simulink model "FRNmodel"  (Simulink 7.9)
settings: Solver=VariableStepDiscrete  StartTime=0.0  StopTime=100.0  RelTol=1e-3
libraries: simeventslib x22, FRN_Library x11
(part 1 of 2)
settings Model: Creator=tsprock3  LastModifiedBy=tsprock3
settings DebuggingCC: SimStateOlderReleaseMsg=warning

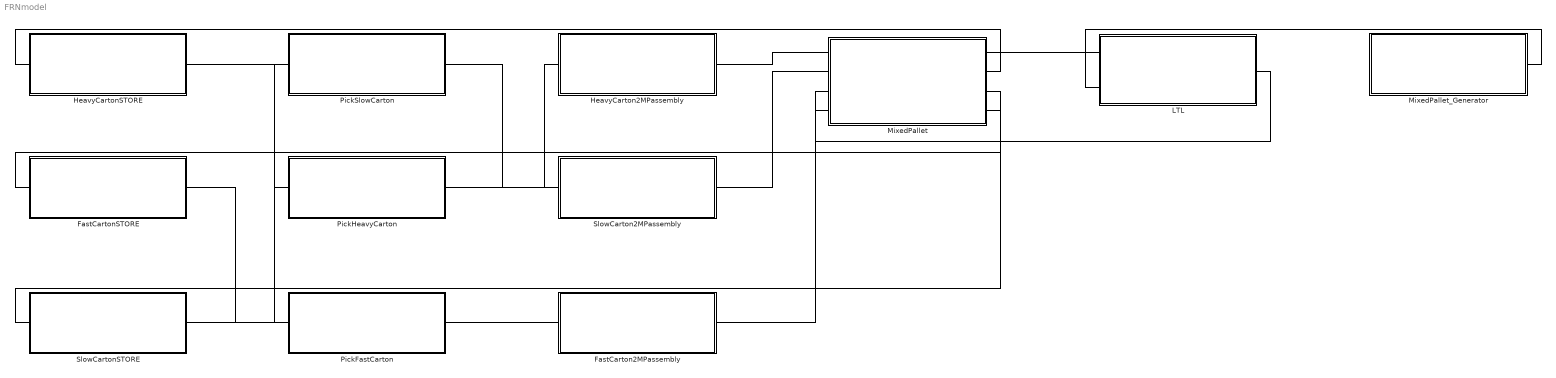
== system FRNmodel ==
  FastCarton2MPassembly : Subsystem
  FastCartonSTORE : Subsystem
  HeavyCarton2MPassembly : Subsystem
  HeavyCartonSTORE : Subsystem
  LTL : Subsystem
  MixedPallet : Subsystem
  MixedPallet_Generator : Subsystem
  PickFastCarton : Subsystem
  PickHeavyCarton : Subsystem
  PickSlowCarton : Subsystem
  SlowCarton2MPassembly : Subsystem
  SlowCartonSTORE : Subsystem
  connections:
  FastCartonSTORE/RConn1 -- PickFastCarton/LConn1
  PickFastCarton/RConn1 -- FastCarton2MPassembly/LConn1
  HeavyCarton2MPassembly/RConn1 -- MixedPallet/LConn1
  MixedPallet/RConn1 -- LTL/LConn1
  PickSlowCarton/RConn1 -- SlowCarton2MPassembly/LConn1
  SlowCarton2MPassembly/RConn1 -- MixedPallet/LConn2
  SlowCartonSTORE/RConn1 -- PickSlowCarton/LConn1
  HeavyCartonSTORE/RConn1 -- PickHeavyCarton/LConn1
  FastCarton2MPassembly/RConn1 -- MixedPallet/LConn3
  PickHeavyCarton/RConn1 -- HeavyCarton2MPassembly/LConn1
  LTL/RConn1 -- MixedPallet/LConn4
  MixedPallet/RConn2 -- HeavyCartonSTORE/LConn1
  MixedPallet/RConn3 -- FastCartonSTORE/LConn1
  MixedPallet/RConn4 -- SlowCartonSTORE/LConn1
  MixedPallet_Generator/RConn1 -- LTL/LConn2

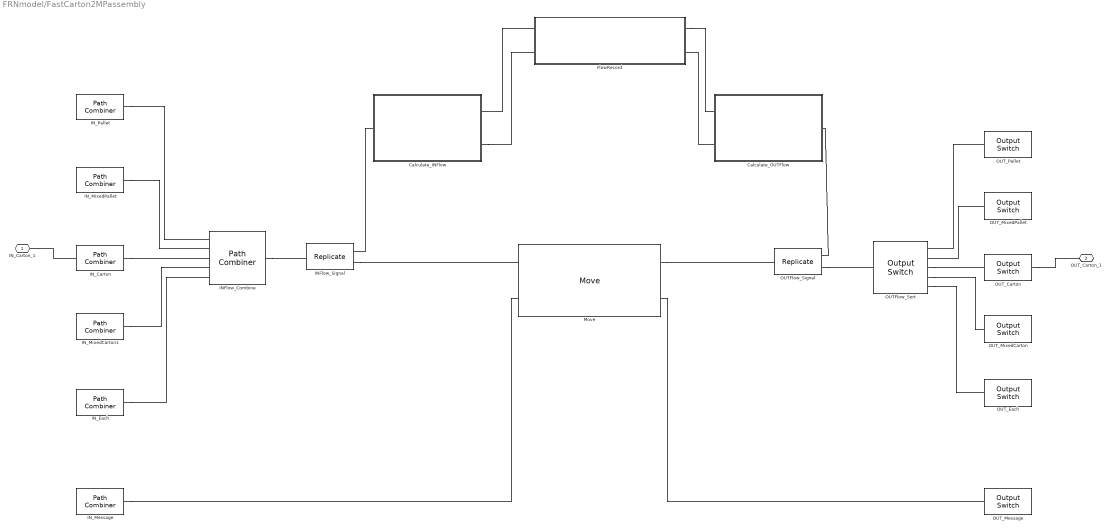
== system FRNmodel/FastCarton2MPassembly ==
  Calculate_INFlow : Subsystem
  Calculate_OUTFlow : Subsystem
  FlowRecord : Subsystem
  INFlow_Combine : PathCombiner  NumberInputPorts=5
  INFlow_Signal : Replicate  NumberOutputPorts=2
  IN_Carton : PathCombiner  NumberInputPorts=1
  IN_Each : PathCombiner  NumberInputPorts=1
  IN_Message : PathCombiner  NumberInputPorts=1
  IN_MixedCarton1 : PathCombiner  NumberInputPorts=1
  IN_MixedPallet : PathCombiner  NumberInputPorts=1
  IN_Pallet : PathCombiner  NumberInputPorts=1
  Move : FRN_Library/Move
  OUTFlow_Signal : Replicate  NumberOutputPorts=2
  OUTFlow_Sort : OutputSwitch  NumberOutputPorts=5  SwitchingCriterion=From attribute  AttributeName=UoH
  OUT_Carton : OutputSwitch  NumberOutputPorts=1
  OUT_Each : OutputSwitch  NumberOutputPorts=1
  OUT_Message : OutputSwitch  NumberOutputPorts=1  SwitchingCriterion=Equiprobable  AttributeName=FlowSource
  OUT_MixedCarton : OutputSwitch  NumberOutputPorts=1
  OUT_MixedPallet : OutputSwitch  NumberOutputPorts=1
  OUT_Pallet : OutputSwitch  NumberOutputPorts=1
  IN_Carton_1 : PMIOPort  Port=1  Side=Left
  OUT_Carton_1 : PMIOPort  Port=2  Side=Right
  connections:
  INFlow_Signal/RConn2 -- Move/LConn1
  IN_MixedCarton1/RConn1 -- INFlow_Combine/LConn4
  IN_MixedPallet/RConn1 -- INFlow_Combine/LConn2
  OUTFlow_Sort/RConn4 -- OUT_MixedCarton/LConn1
  OUT_MixedPallet/LConn1 -- OUTFlow_Sort/RConn2
  Move/RConn2 -- OUT_Message/LConn1
  IN_Message/RConn1 -- Move/LConn2
  OUTFlow_Sort/RConn5 -- OUT_Each/LConn1
  OUTFlow_Sort/RConn3 -- OUT_Carton/LConn1
  OUT_Pallet/LConn1 -- OUTFlow_Sort/RConn1
  OUTFlow_Signal/RConn2 -- OUTFlow_Sort/LConn1
  IN_Each/RConn1 -- INFlow_Combine/LConn5
  IN_Carton/RConn1 -- INFlow_Combine/LConn3
  IN_Pallet/RConn1 -- INFlow_Combine/LConn1
  INFlow_Combine/RConn1 -- INFlow_Signal/LConn1
  OUTFlow_Signal/RConn1 -- Calculate_OUTFlow/RConn1
  Move/RConn1 -- OUTFlow_Signal/LConn1
  Calculate_OUTFlow/LConn2 -- FlowRecord/LConn2
  FlowRecord/LConn1 -- Calculate_OUTFlow/LConn1
  Calculate_INFlow/RConn2 -- FlowRecord/RConn2
  FlowRecord/RConn1 -- Calculate_INFlow/RConn1
  Calculate_INFlow/LConn1 -- INFlow_Signal/RConn1
  IN_Carton/LConn1 -- IN_Carton_1/RConn1
  OUT_Carton/RConn1 -- OUT_Carton_1/RConn1

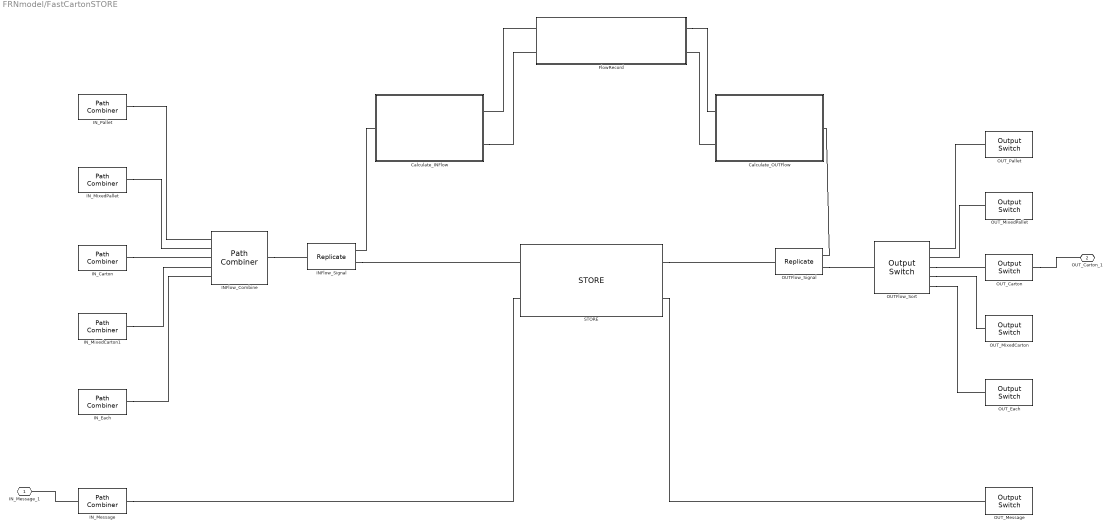
== system FRNmodel/FastCartonSTORE ==
  Calculate_INFlow : Subsystem
  Calculate_OUTFlow : Subsystem
  FlowRecord : Subsystem
  INFlow_Combine : PathCombiner  NumberInputPorts=5
  INFlow_Signal : Replicate  NumberOutputPorts=2
  IN_Carton : PathCombiner  NumberInputPorts=1
  IN_Each : PathCombiner  NumberInputPorts=1
  IN_Message : PathCombiner  NumberInputPorts=1
  IN_MixedCarton1 : PathCombiner  NumberInputPorts=1
  IN_MixedPallet : PathCombiner  NumberInputPorts=1
  IN_Pallet : PathCombiner  NumberInputPorts=1
  OUTFlow_Signal : Replicate  NumberOutputPorts=2
  OUTFlow_Sort : OutputSwitch  NumberOutputPorts=5  SwitchingCriterion=From attribute  AttributeName=UoH
  OUT_Carton : OutputSwitch  NumberOutputPorts=1
  OUT_Each : OutputSwitch  NumberOutputPorts=1
  OUT_Message : OutputSwitch  NumberOutputPorts=1  SwitchingCriterion=Equiprobable  AttributeName=FlowSource
  OUT_MixedCarton : OutputSwitch  NumberOutputPorts=1
  OUT_MixedPallet : OutputSwitch  NumberOutputPorts=1
  OUT_Pallet : OutputSwitch  NumberOutputPorts=1
  STORE : FRN_Library/STORE
  IN_Message_1 : PMIOPort  Port=1  Side=Left
  OUT_Carton_1 : PMIOPort  Port=2  Side=Right
  connections:
  INFlow_Signal/RConn2 -- STORE/LConn1
  IN_MixedCarton1/RConn1 -- INFlow_Combine/LConn4
  IN_MixedPallet/RConn1 -- INFlow_Combine/LConn2
  OUTFlow_Sort/RConn4 -- OUT_MixedCarton/LConn1
  OUT_MixedPallet/LConn1 -- OUTFlow_Sort/RConn2
  STORE/RConn2 -- OUT_Message/LConn1
  IN_Message/RConn1 -- STORE/LConn2
  OUTFlow_Sort/RConn5 -- OUT_Each/LConn1
  OUTFlow_Sort/RConn3 -- OUT_Carton/LConn1
  OUT_Pallet/LConn1 -- OUTFlow_Sort/RConn1
  OUTFlow_Signal/RConn2 -- OUTFlow_Sort/LConn1
  IN_Each/RConn1 -- INFlow_Combine/LConn5
  IN_Carton/RConn1 -- INFlow_Combine/LConn3
  IN_Pallet/RConn1 -- INFlow_Combine/LConn1
  INFlow_Combine/RConn1 -- INFlow_Signal/LConn1
  OUTFlow_Signal/RConn1 -- Calculate_OUTFlow/RConn1
  STORE/RConn1 -- OUTFlow_Signal/LConn1
  Calculate_OUTFlow/LConn2 -- FlowRecord/LConn2
  FlowRecord/LConn1 -- Calculate_OUTFlow/LConn1
  Calculate_INFlow/RConn2 -- FlowRecord/RConn2
  FlowRecord/RConn1 -- Calculate_INFlow/RConn1
  Calculate_INFlow/LConn1 -- INFlow_Signal/RConn1
  IN_Message/LConn1 -- IN_Message_1/RConn1
  OUT_Carton/RConn1 -- OUT_Carton_1/RConn1

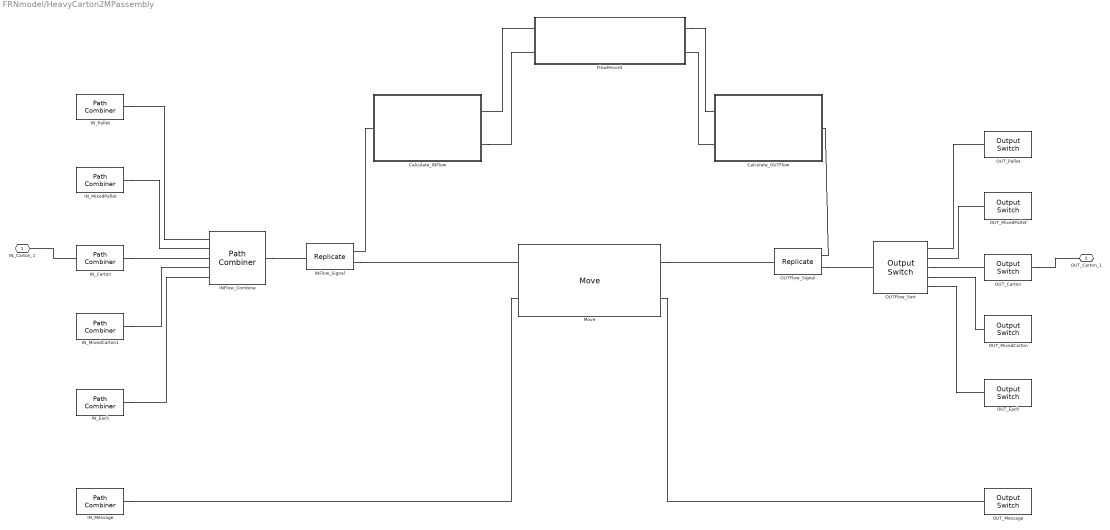
== system FRNmodel/HeavyCarton2MPassembly ==
  Calculate_INFlow : Subsystem
  Calculate_OUTFlow : Subsystem
  FlowRecord : Subsystem
  INFlow_Combine : PathCombiner  NumberInputPorts=5
  INFlow_Signal : Replicate  NumberOutputPorts=2
  IN_Carton : PathCombiner  NumberInputPorts=1
  IN_Each : PathCombiner  NumberInputPorts=1
  IN_Message : PathCombiner  NumberInputPorts=1
  IN_MixedCarton1 : PathCombiner  NumberInputPorts=1
  IN_MixedPallet : PathCombiner  NumberInputPorts=1
  IN_Pallet : PathCombiner  NumberInputPorts=1
  Move : FRN_Library/Move
  OUTFlow_Signal : Replicate  NumberOutputPorts=2
  OUTFlow_Sort : OutputSwitch  NumberOutputPorts=5  SwitchingCriterion=From attribute  AttributeName=UoH
  OUT_Carton : OutputSwitch  NumberOutputPorts=1
  OUT_Each : OutputSwitch  NumberOutputPorts=1
  OUT_Message : OutputSwitch  NumberOutputPorts=1  SwitchingCriterion=Equiprobable  AttributeName=FlowSource
  OUT_MixedCarton : OutputSwitch  NumberOutputPorts=1
  OUT_MixedPallet : OutputSwitch  NumberOutputPorts=1
  OUT_Pallet : OutputSwitch  NumberOutputPorts=1
  IN_Carton_1 : PMIOPort  Port=1  Side=Left
  OUT_Carton_1 : PMIOPort  Port=2  Side=Right
  connections:
  INFlow_Signal/RConn2 -- Move/LConn1
  IN_MixedCarton1/RConn1 -- INFlow_Combine/LConn4
  IN_MixedPallet/RConn1 -- INFlow_Combine/LConn2
  OUTFlow_Sort/RConn4 -- OUT_MixedCarton/LConn1
  OUT_MixedPallet/LConn1 -- OUTFlow_Sort/RConn2
  Move/RConn2 -- OUT_Message/LConn1
  IN_Message/RConn1 -- Move/LConn2
  OUTFlow_Sort/RConn5 -- OUT_Each/LConn1
  OUTFlow_Sort/RConn3 -- OUT_Carton/LConn1
  OUT_Pallet/LConn1 -- OUTFlow_Sort/RConn1
  OUTFlow_Signal/RConn2 -- OUTFlow_Sort/LConn1
  IN_Each/RConn1 -- INFlow_Combine/LConn5
  IN_Carton/RConn1 -- INFlow_Combine/LConn3
  IN_Pallet/RConn1 -- INFlow_Combine/LConn1
  INFlow_Combine/RConn1 -- INFlow_Signal/LConn1
  OUTFlow_Signal/RConn1 -- Calculate_OUTFlow/RConn1
  Move/RConn1 -- OUTFlow_Signal/LConn1
  Calculate_OUTFlow/LConn2 -- FlowRecord/LConn2
  FlowRecord/LConn1 -- Calculate_OUTFlow/LConn1
  Calculate_INFlow/RConn2 -- FlowRecord/RConn2
  FlowRecord/RConn1 -- Calculate_INFlow/RConn1
  Calculate_INFlow/LConn1 -- INFlow_Signal/RConn1
  IN_Carton/LConn1 -- IN_Carton_1/RConn1
  OUT_Carton/RConn1 -- OUT_Carton_1/RConn1

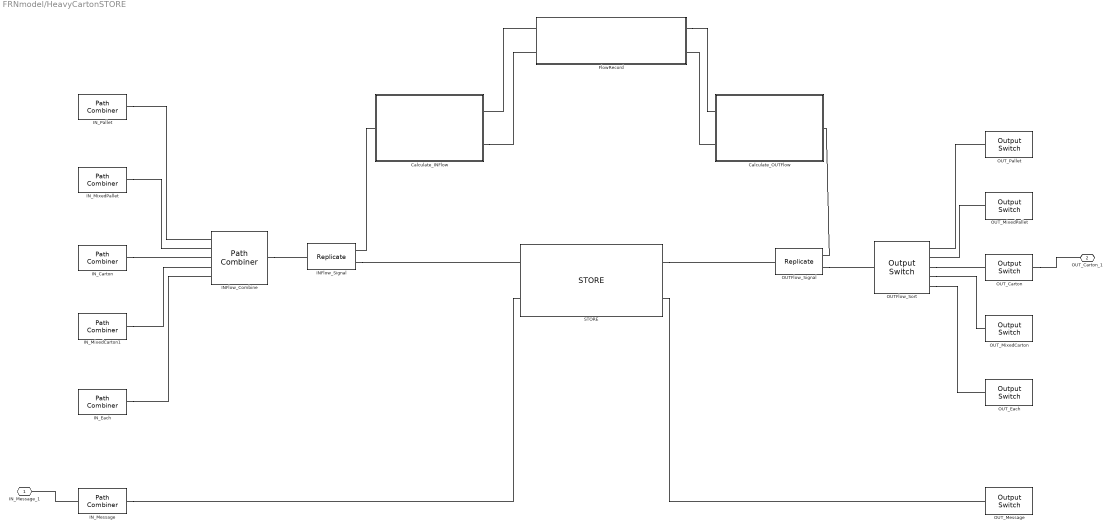
== system FRNmodel/HeavyCartonSTORE ==
  Calculate_INFlow : Subsystem
  Calculate_OUTFlow : Subsystem
  FlowRecord : Subsystem
  INFlow_Combine : PathCombiner  NumberInputPorts=5
  INFlow_Signal : Replicate  NumberOutputPorts=2
  IN_Carton : PathCombiner  NumberInputPorts=1
  IN_Each : PathCombiner  NumberInputPorts=1
  IN_Message : PathCombiner  NumberInputPorts=1
  IN_MixedCarton1 : PathCombiner  NumberInputPorts=1
  IN_MixedPallet : PathCombiner  NumberInputPorts=1
  IN_Pallet : PathCombiner  NumberInputPorts=1
  OUTFlow_Signal : Replicate  NumberOutputPorts=2
  OUTFlow_Sort : OutputSwitch  NumberOutputPorts=5  SwitchingCriterion=From attribute  AttributeName=UoH
  OUT_Carton : OutputSwitch  NumberOutputPorts=1
  OUT_Each : OutputSwitch  NumberOutputPorts=1
  OUT_Message : OutputSwitch  NumberOutputPorts=1  SwitchingCriterion=Equiprobable  AttributeName=FlowSource
  OUT_MixedCarton : OutputSwitch  NumberOutputPorts=1
  OUT_MixedPallet : OutputSwitch  NumberOutputPorts=1
  OUT_Pallet : OutputSwitch  NumberOutputPorts=1
  STORE : FRN_Library/STORE
  IN_Message_1 : PMIOPort  Port=1  Side=Left
  OUT_Carton_1 : PMIOPort  Port=2  Side=Right
  connections:
  INFlow_Signal/RConn2 -- STORE/LConn1
  IN_MixedCarton1/RConn1 -- INFlow_Combine/LConn4
  IN_MixedPallet/RConn1 -- INFlow_Combine/LConn2
  OUTFlow_Sort/RConn4 -- OUT_MixedCarton/LConn1
  OUT_MixedPallet/LConn1 -- OUTFlow_Sort/RConn2
  STORE/RConn2 -- OUT_Message/LConn1
  IN_Message/RConn1 -- STORE/LConn2
  OUTFlow_Sort/RConn5 -- OUT_Each/LConn1
  OUTFlow_Sort/RConn3 -- OUT_Carton/LConn1
  OUT_Pallet/LConn1 -- OUTFlow_Sort/RConn1
  OUTFlow_Signal/RConn2 -- OUTFlow_Sort/LConn1
  IN_Each/RConn1 -- INFlow_Combine/LConn5
  IN_Carton/RConn1 -- INFlow_Combine/LConn3
  IN_Pallet/RConn1 -- INFlow_Combine/LConn1
  INFlow_Combine/RConn1 -- INFlow_Signal/LConn1
  OUTFlow_Signal/RConn1 -- Calculate_OUTFlow/RConn1
  STORE/RConn1 -- OUTFlow_Signal/LConn1
  Calculate_OUTFlow/LConn2 -- FlowRecord/LConn2
  FlowRecord/LConn1 -- Calculate_OUTFlow/LConn1
  Calculate_INFlow/RConn2 -- FlowRecord/RConn2
  FlowRecord/RConn1 -- Calculate_INFlow/RConn1
  Calculate_INFlow/LConn1 -- INFlow_Signal/RConn1
  IN_Message/LConn1 -- IN_Message_1/RConn1
  OUT_Carton/RConn1 -- OUT_Carton_1/RConn1

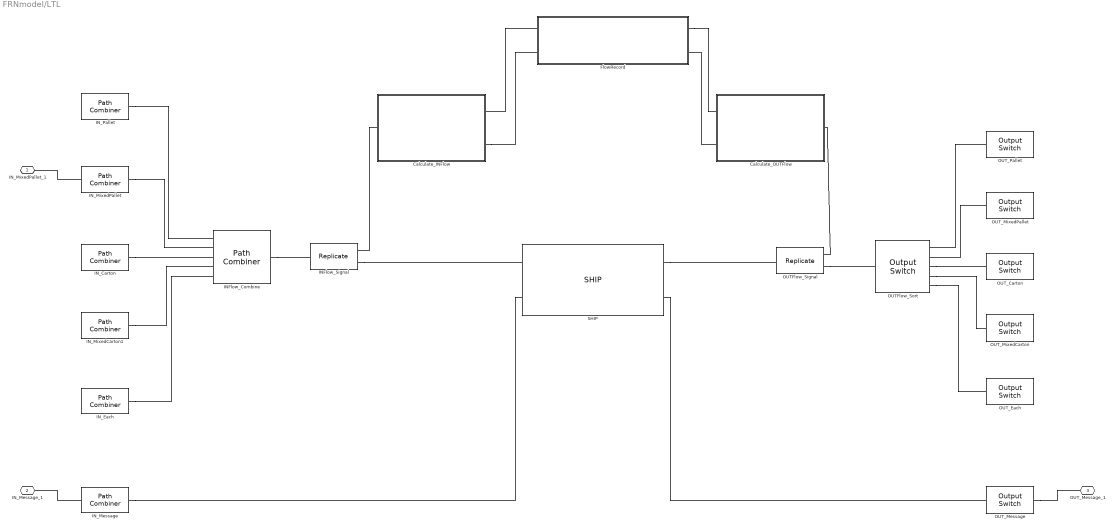
== system FRNmodel/LTL ==
  Calculate_INFlow : Subsystem
  Calculate_OUTFlow : Subsystem
  FlowRecord : Subsystem
  INFlow_Combine : PathCombiner  NumberInputPorts=5
  INFlow_Signal : Replicate  NumberOutputPorts=2
  IN_Carton : PathCombiner  NumberInputPorts=1
  IN_Each : PathCombiner  NumberInputPorts=1
  IN_Message : PathCombiner  NumberInputPorts=1
  IN_MixedCarton1 : PathCombiner  NumberInputPorts=1
  IN_MixedPallet : PathCombiner  NumberInputPorts=1
  IN_Pallet : PathCombiner  NumberInputPorts=1
  OUTFlow_Signal : Replicate  NumberOutputPorts=2
  OUTFlow_Sort : OutputSwitch  NumberOutputPorts=5  SwitchingCriterion=From attribute  AttributeName=UoH
  OUT_Carton : OutputSwitch  NumberOutputPorts=1
  OUT_Each : OutputSwitch  NumberOutputPorts=1
  OUT_Message : OutputSwitch  NumberOutputPorts=1  SwitchingCriterion=Equiprobable  AttributeName=FlowSource
  OUT_MixedCarton : OutputSwitch  NumberOutputPorts=1
  OUT_MixedPallet : OutputSwitch  NumberOutputPorts=1
  OUT_Pallet : OutputSwitch  NumberOutputPorts=1
  SHIP : FRN_Library/SHIP
  IN_MixedPallet_1 : PMIOPort  Port=1  Side=Left
  IN_Message_1 : PMIOPort  Port=2  Side=Left
  OUT_Message_1 : PMIOPort  Port=3  Side=Right
  connections:
  INFlow_Signal/RConn2 -- SHIP/LConn1
  IN_MixedCarton1/RConn1 -- INFlow_Combine/LConn4
  IN_MixedPallet/RConn1 -- INFlow_Combine/LConn2
  OUTFlow_Sort/RConn4 -- OUT_MixedCarton/LConn1
  OUT_MixedPallet/LConn1 -- OUTFlow_Sort/RConn2
  SHIP/RConn2 -- OUT_Message/LConn1
  IN_Message/RConn1 -- SHIP/LConn2
  OUTFlow_Sort/RConn5 -- OUT_Each/LConn1
  OUTFlow_Sort/RConn3 -- OUT_Carton/LConn1
  OUT_Pallet/LConn1 -- OUTFlow_Sort/RConn1
  OUTFlow_Signal/RConn2 -- OUTFlow_Sort/LConn1
  IN_Each/RConn1 -- INFlow_Combine/LConn5
  IN_Carton/RConn1 -- INFlow_Combine/LConn3
  IN_Pallet/RConn1 -- INFlow_Combine/LConn1
  INFlow_Combine/RConn1 -- INFlow_Signal/LConn1
  OUTFlow_Signal/RConn1 -- Calculate_OUTFlow/RConn1
  SHIP/RConn1 -- OUTFlow_Signal/LConn1
  Calculate_OUTFlow/LConn2 -- FlowRecord/LConn2
  FlowRecord/LConn1 -- Calculate_OUTFlow/LConn1
  Calculate_INFlow/RConn2 -- FlowRecord/RConn2
  FlowRecord/RConn1 -- Calculate_INFlow/RConn1
  Calculate_INFlow/LConn1 -- INFlow_Signal/RConn1
  IN_MixedPallet/LConn1 -- IN_MixedPallet_1/RConn1
  IN_Message/LConn1 -- IN_Message_1/RConn1
  OUT_Message/RConn1 -- OUT_Message_1/RConn1

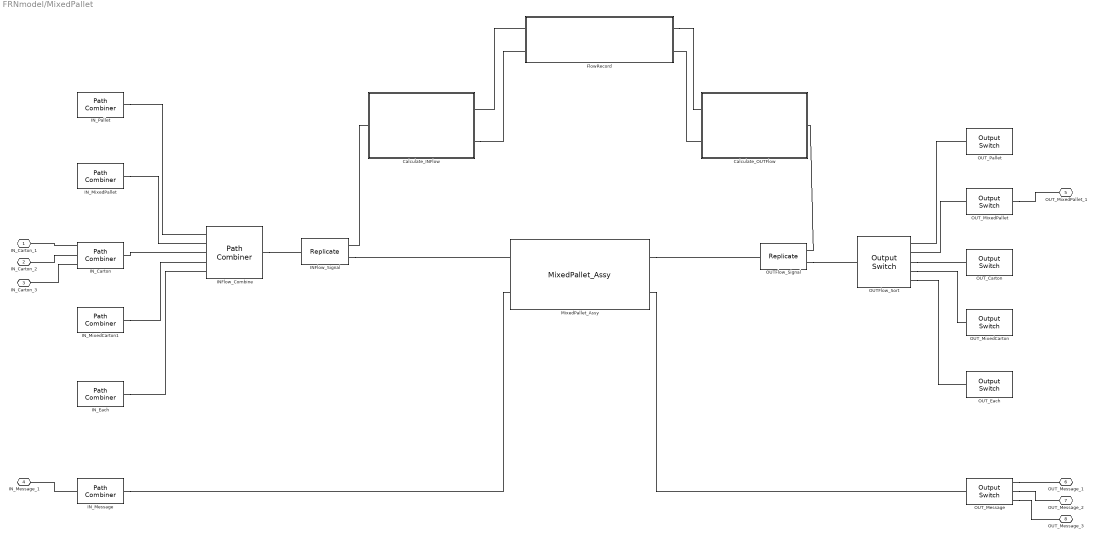
== system FRNmodel/MixedPallet ==
  Calculate_INFlow : Subsystem
  Calculate_OUTFlow : Subsystem
  FlowRecord : Subsystem
  INFlow_Combine : PathCombiner  NumberInputPorts=5
  INFlow_Signal : Replicate  NumberOutputPorts=2
  IN_Carton : PathCombiner
  IN_Each : PathCombiner  NumberInputPorts=1
  IN_Message : PathCombiner  NumberInputPorts=1
  IN_MixedCarton1 : PathCombiner  NumberInputPorts=1
  IN_MixedPallet : PathCombiner  NumberInputPorts=1
  IN_Pallet : PathCombiner  NumberInputPorts=1
  MixedPallet_Assy : FRN_Library/MixedPallet_Assy
  OUTFlow_Signal : Replicate  NumberOutputPorts=2
  OUTFlow_Sort : OutputSwitch  NumberOutputPorts=5  SwitchingCriterion=From attribute  AttributeName=UoH
  OUT_Carton : OutputSwitch  NumberOutputPorts=1
  OUT_Each : OutputSwitch  NumberOutputPorts=1
  OUT_Message : OutputSwitch  SwitchingCriterion=Equiprobable  AttributeName=FlowSource
  OUT_MixedCarton : OutputSwitch  NumberOutputPorts=1
  OUT_MixedPallet : OutputSwitch  NumberOutputPorts=1
  OUT_Pallet : OutputSwitch  NumberOutputPorts=1
  IN_Carton_1 : PMIOPort  Port=1  Side=Left
  IN_Carton_2 : PMIOPort  Port=2  Side=Left
  IN_Carton_3 : PMIOPort  Port=3  Side=Left
  IN_Message_1 : PMIOPort  Port=4  Side=Left
  OUT_MixedPallet_1 : PMIOPort  Port=5  Side=Right
  OUT_Message_1 : PMIOPort  Port=6  Side=Right
  OUT_Message_2 : PMIOPort  Port=7  Side=Right
  OUT_Message_3 : PMIOPort  Port=8  Side=Right
  connections:
  INFlow_Signal/RConn2 -- MixedPallet_Assy/LConn1
  IN_MixedCarton1/RConn1 -- INFlow_Combine/LConn4
  IN_MixedPallet/RConn1 -- INFlow_Combine/LConn2
  OUTFlow_Sort/RConn4 -- OUT_MixedCarton/LConn1
  OUT_MixedPallet/LConn1 -- OUTFlow_Sort/RConn2
  MixedPallet_Assy/RConn2 -- OUT_Message/LConn1
  IN_Message/RConn1 -- MixedPallet_Assy/LConn2
  OUTFlow_Sort/RConn5 -- OUT_Each/LConn1
  OUTFlow_Sort/RConn3 -- OUT_Carton/LConn1
  OUT_Pallet/LConn1 -- OUTFlow_Sort/RConn1
  OUTFlow_Signal/RConn2 -- OUTFlow_Sort/LConn1
  IN_Each/RConn1 -- INFlow_Combine/LConn5
  IN_Carton/RConn1 -- INFlow_Combine/LConn3
  IN_Pallet/RConn1 -- INFlow_Combine/LConn1
  INFlow_Combine/RConn1 -- INFlow_Signal/LConn1
  OUTFlow_Signal/RConn1 -- Calculate_OUTFlow/RConn1
  MixedPallet_Assy/RConn1 -- OUTFlow_Signal/LConn1
  Calculate_OUTFlow/LConn2 -- FlowRecord/LConn2
  FlowRecord/LConn1 -- Calculate_OUTFlow/LConn1
  Calculate_INFlow/RConn2 -- FlowRecord/RConn2
  FlowRecord/RConn1 -- Calculate_INFlow/RConn1
  Calculate_INFlow/LConn1 -- INFlow_Signal/RConn1
  IN_Carton/LConn1 -- IN_Carton_1/RConn1
  IN_Carton/LConn2 -- IN_Carton_2/RConn1
  IN_Carton/LConn3 -- IN_Carton_3/RConn1
  IN_Message/LConn1 -- IN_Message_1/RConn1
  OUT_MixedPallet/RConn1 -- OUT_MixedPallet_1/RConn1
  OUT_Message/RConn1 -- OUT_Message_1/RConn1
  OUT_Message/RConn2 -- OUT_Message_2/RConn1
  OUT_Message/RConn3 -- OUT_Message_3/RConn1

== system FRNmodel/MixedPallet_Generator ==
  OUT_Message : OutputSwitch  NumberOutputPorts=1
  Set Attribute : SetAttribute  AttributeName=UoH|CartonQuantity  AttributeFrom=Dialog|Dialog  AttributeValue=3|100  AttributeTreatAsVector=1|1  EvaluatedAttributeValue={3;100}
  Time-Based Entity Generator : TimeBasedEntityGenerator
  OUT_Message_1 : PMIOPort  Port=1  Side=Right
  connections:
  Set Attribute/RConn1 -- OUT_Message/LConn1
  Time-Based Entity Generator/RConn1 -- Set Attribute/LConn1
  OUT_Message/RConn1 -- OUT_Message_1/RConn1

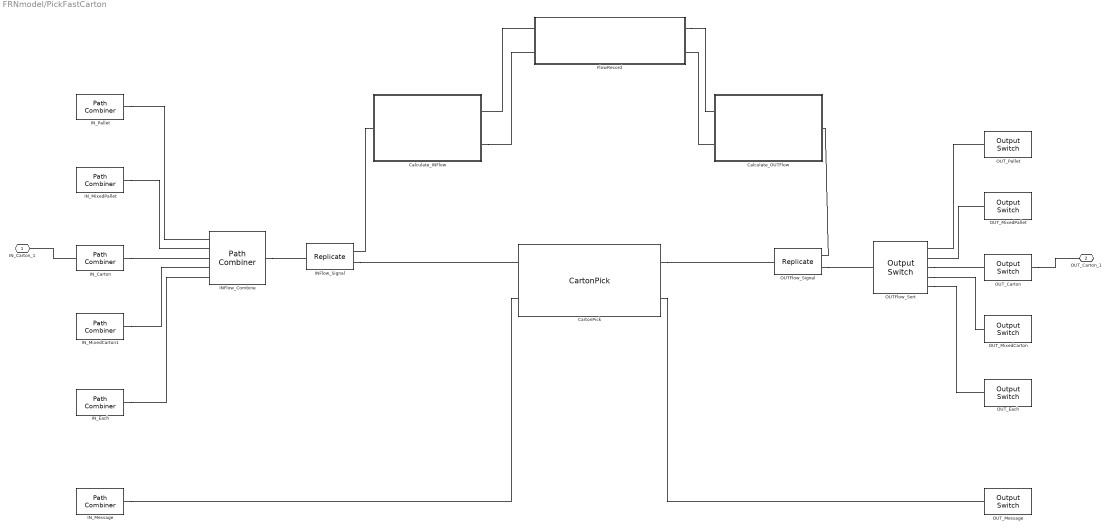
== system FRNmodel/PickFastCarton ==
  Calculate_INFlow : Subsystem
  Calculate_OUTFlow : Subsystem
  CartonPick : FRN_Library/CartonPick
  FlowRecord : Subsystem
  INFlow_Combine : PathCombiner  NumberInputPorts=5
  INFlow_Signal : Replicate  NumberOutputPorts=2
  IN_Carton : PathCombiner  NumberInputPorts=1
  IN_Each : PathCombiner  NumberInputPorts=1
  IN_Message : PathCombiner  NumberInputPorts=1
  IN_MixedCarton1 : PathCombiner  NumberInputPorts=1
  IN_MixedPallet : PathCombiner  NumberInputPorts=1
  IN_Pallet : PathCombiner  NumberInputPorts=1
  OUTFlow_Signal : Replicate  NumberOutputPorts=2
  OUTFlow_Sort : OutputSwitch  NumberOutputPorts=5  SwitchingCriterion=From attribute  AttributeName=UoH
  OUT_Carton : OutputSwitch  NumberOutputPorts=1
  OUT_Each : OutputSwitch  NumberOutputPorts=1
  OUT_Message : OutputSwitch  NumberOutputPorts=1  SwitchingCriterion=Equiprobable  AttributeName=FlowSource
  OUT_MixedCarton : OutputSwitch  NumberOutputPorts=1
  OUT_MixedPallet : OutputSwitch  NumberOutputPorts=1
  OUT_Pallet : OutputSwitch  NumberOutputPorts=1
  IN_Carton_1 : PMIOPort  Port=1  Side=Left
  OUT_Carton_1 : PMIOPort  Port=2  Side=Right
  connections:
  INFlow_Signal/RConn2 -- CartonPick/LConn1
  IN_MixedCarton1/RConn1 -- INFlow_Combine/LConn4
  IN_MixedPallet/RConn1 -- INFlow_Combine/LConn2
  OUTFlow_Sort/RConn4 -- OUT_MixedCarton/LConn1
  OUT_MixedPallet/LConn1 -- OUTFlow_Sort/RConn2
  CartonPick/RConn2 -- OUT_Message/LConn1
  IN_Message/RConn1 -- CartonPick/LConn2
  OUTFlow_Sort/RConn5 -- OUT_Each/LConn1
  OUTFlow_Sort/RConn3 -- OUT_Carton/LConn1
  OUT_Pallet/LConn1 -- OUTFlow_Sort/RConn1
  OUTFlow_Signal/RConn2 -- OUTFlow_Sort/LConn1
  IN_Each/RConn1 -- INFlow_Combine/LConn5
  IN_Carton/RConn1 -- INFlow_Combine/LConn3
  IN_Pallet/RConn1 -- INFlow_Combine/LConn1
  INFlow_Combine/RConn1 -- INFlow_Signal/LConn1
  OUTFlow_Signal/RConn1 -- Calculate_OUTFlow/RConn1
  CartonPick/RConn1 -- OUTFlow_Signal/LConn1
  Calculate_OUTFlow/LConn2 -- FlowRecord/LConn2
  FlowRecord/LConn1 -- Calculate_OUTFlow/LConn1
  Calculate_INFlow/RConn2 -- FlowRecord/RConn2
  FlowRecord/RConn1 -- Calculate_INFlow/RConn1
  Calculate_INFlow/LConn1 -- INFlow_Signal/RConn1
  IN_Carton/LConn1 -- IN_Carton_1/RConn1
  OUT_Carton/RConn1 -- OUT_Carton_1/RConn1

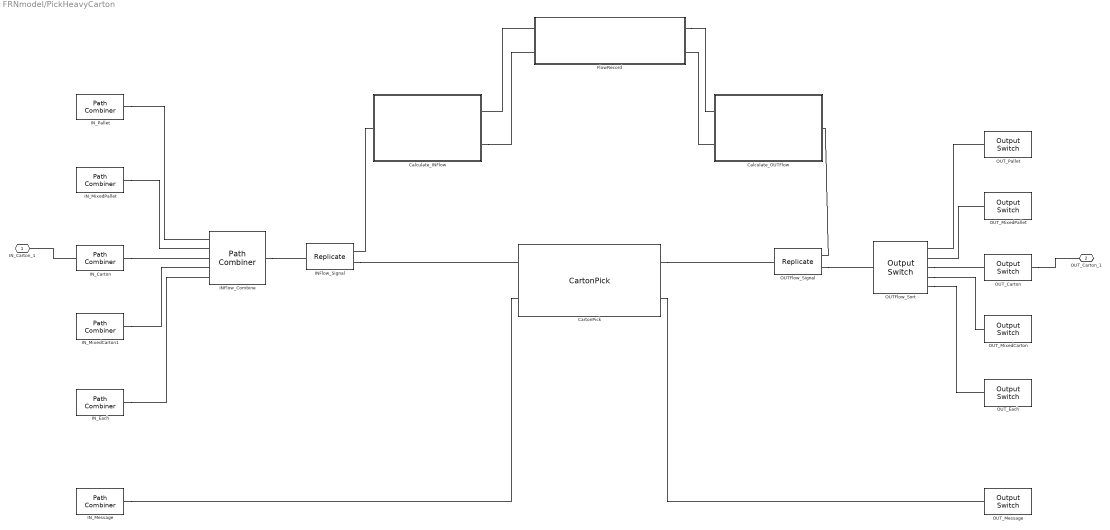
== system FRNmodel/PickHeavyCarton ==
  Calculate_INFlow : Subsystem
  Calculate_OUTFlow : Subsystem
  CartonPick : FRN_Library/CartonPick
  FlowRecord : Subsystem
  INFlow_Combine : PathCombiner  NumberInputPorts=5
  INFlow_Signal : Replicate  NumberOutputPorts=2
  IN_Carton : PathCombiner  NumberInputPorts=1
  IN_Each : PathCombiner  NumberInputPorts=1
  IN_Message : PathCombiner  NumberInputPorts=1
  IN_MixedCarton1 : PathCombiner  NumberInputPorts=1
  IN_MixedPallet : PathCombiner  NumberInputPorts=1
  IN_Pallet : PathCombiner  NumberInputPorts=1
  OUTFlow_Signal : Replicate  NumberOutputPorts=2
  OUTFlow_Sort : OutputSwitch  NumberOutputPorts=5  SwitchingCriterion=From attribute  AttributeName=UoH
  OUT_Carton : OutputSwitch  NumberOutputPorts=1
  OUT_Each : OutputSwitch  NumberOutputPorts=1
  OUT_Message : OutputSwitch  NumberOutputPorts=1  SwitchingCriterion=Equiprobable  AttributeName=FlowSource
  OUT_MixedCarton : OutputSwitch  NumberOutputPorts=1
  OUT_MixedPallet : OutputSwitch  NumberOutputPorts=1
  OUT_Pallet : OutputSwitch  NumberOutputPorts=1
  IN_Carton_1 : PMIOPort  Port=1  Side=Left
  OUT_Carton_1 : PMIOPort  Port=2  Side=Right
  connections:
  INFlow_Signal/RConn2 -- CartonPick/LConn1
  IN_MixedCarton1/RConn1 -- INFlow_Combine/LConn4
  IN_MixedPallet/RConn1 -- INFlow_Combine/LConn2
  OUTFlow_Sort/RConn4 -- OUT_MixedCarton/LConn1
  OUT_MixedPallet/LConn1 -- OUTFlow_Sort/RConn2
  CartonPick/RConn2 -- OUT_Message/LConn1
  IN_Message/RConn1 -- CartonPick/LConn2
  OUTFlow_Sort/RConn5 -- OUT_Each/LConn1
  OUTFlow_Sort/RConn3 -- OUT_Carton/LConn1
  OUT_Pallet/LConn1 -- OUTFlow_Sort/RConn1
  OUTFlow_Signal/RConn2 -- OUTFlow_Sort/LConn1
  IN_Each/RConn1 -- INFlow_Combine/LConn5
  IN_Carton/RConn1 -- INFlow_Combine/LConn3
  IN_Pallet/RConn1 -- INFlow_Combine/LConn1
  INFlow_Combine/RConn1 -- INFlow_Signal/LConn1
  OUTFlow_Signal/RConn1 -- Calculate_OUTFlow/RConn1
  CartonPick/RConn1 -- OUTFlow_Signal/LConn1
  Calculate_OUTFlow/LConn2 -- FlowRecord/LConn2
  FlowRecord/LConn1 -- Calculate_OUTFlow/LConn1
  Calculate_INFlow/RConn2 -- FlowRecord/RConn2
  FlowRecord/RConn1 -- Calculate_INFlow/RConn1
  Calculate_INFlow/LConn1 -- INFlow_Signal/RConn1
  IN_Carton/LConn1 -- IN_Carton_1/RConn1
  OUT_Carton/RConn1 -- OUT_Carton_1/RConn1

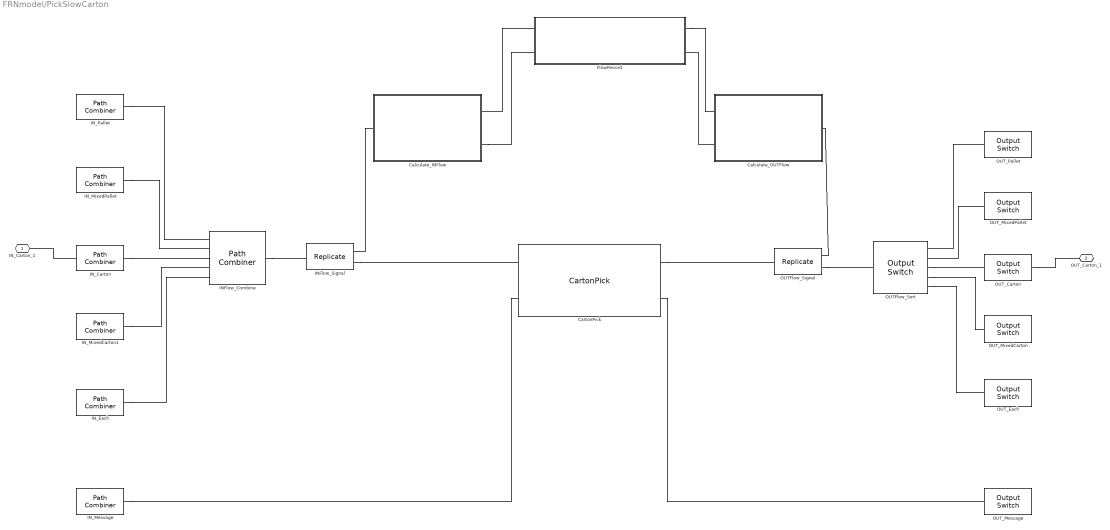
== system FRNmodel/PickSlowCarton ==
  Calculate_INFlow : Subsystem
  Calculate_OUTFlow : Subsystem
  CartonPick : FRN_Library/CartonPick
  FlowRecord : Subsystem
  INFlow_Combine : PathCombiner  NumberInputPorts=5
  INFlow_Signal : Replicate  NumberOutputPorts=2
  IN_Carton : PathCombiner  NumberInputPorts=1
  IN_Each : PathCombiner  NumberInputPorts=1
  IN_Message : PathCombiner  NumberInputPorts=1
  IN_MixedCarton1 : PathCombiner  NumberInputPorts=1
  IN_MixedPallet : PathCombiner  NumberInputPorts=1
  IN_Pallet : PathCombiner  NumberInputPorts=1
  OUTFlow_Signal : Replicate  NumberOutputPorts=2
  OUTFlow_Sort : OutputSwitch  NumberOutputPorts=5  SwitchingCriterion=From attribute  AttributeName=UoH
  OUT_Carton : OutputSwitch  NumberOutputPorts=1
  OUT_Each : OutputSwitch  NumberOutputPorts=1
  OUT_Message : OutputSwitch  NumberOutputPorts=1  SwitchingCriterion=Equiprobable  AttributeName=FlowSource
  OUT_MixedCarton : OutputSwitch  NumberOutputPorts=1
  OUT_MixedPallet : OutputSwitch  NumberOutputPorts=1
  OUT_Pallet : OutputSwitch  NumberOutputPorts=1
  IN_Carton_1 : PMIOPort  Port=1  Side=Left
  OUT_Carton_1 : PMIOPort  Port=2  Side=Right
  connections:
  INFlow_Signal/RConn2 -- CartonPick/LConn1
  IN_MixedCarton1/RConn1 -- INFlow_Combine/LConn4
  IN_MixedPallet/RConn1 -- INFlow_Combine/LConn2
  OUTFlow_Sort/RConn4 -- OUT_MixedCarton/LConn1
  OUT_MixedPallet/LConn1 -- OUTFlow_Sort/RConn2
  CartonPick/RConn2 -- OUT_Message/LConn1
  IN_Message/RConn1 -- CartonPick/LConn2
  OUTFlow_Sort/RConn5 -- OUT_Each/LConn1
  OUTFlow_Sort/RConn3 -- OUT_Carton/LConn1
  OUT_Pallet/LConn1 -- OUTFlow_Sort/RConn1
  OUTFlow_Signal/RConn2 -- OUTFlow_Sort/LConn1
  IN_Each/RConn1 -- INFlow_Combine/LConn5
  IN_Carton/RConn1 -- INFlow_Combine/LConn3
  IN_Pallet/RConn1 -- INFlow_Combine/LConn1
  INFlow_Combine/RConn1 -- INFlow_Signal/LConn1
  OUTFlow_Signal/RConn1 -- Calculate_OUTFlow/RConn1
  CartonPick/RConn1 -- OUTFlow_Signal/LConn1
  Calculate_OUTFlow/LConn2 -- FlowRecord/LConn2
  FlowRecord/LConn1 -- Calculate_OUTFlow/LConn1
  Calculate_INFlow/RConn2 -- FlowRecord/RConn2
  FlowRecord/RConn1 -- Calculate_INFlow/RConn1
  Calculate_INFlow/LConn1 -- INFlow_Signal/RConn1
  IN_Carton/LConn1 -- IN_Carton_1/RConn1
  OUT_Carton/RConn1 -- OUT_Carton_1/RConn1

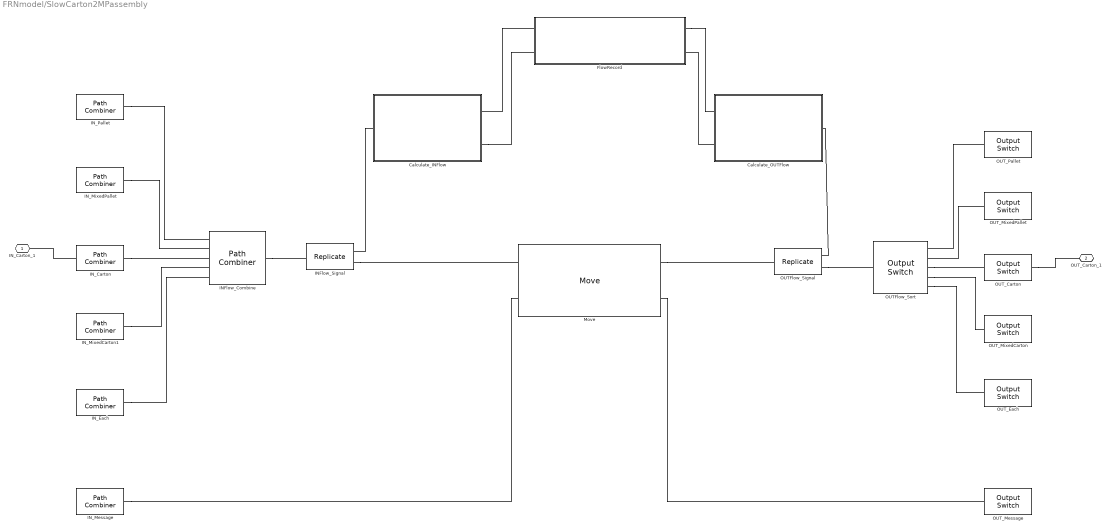
== system FRNmodel/SlowCarton2MPassembly ==
  Calculate_INFlow : Subsystem
  Calculate_OUTFlow : Subsystem
  FlowRecord : Subsystem
  INFlow_Combine : PathCombiner  NumberInputPorts=5
  INFlow_Signal : Replicate  NumberOutputPorts=2
  IN_Carton : PathCombiner  NumberInputPorts=1
  IN_Each : PathCombiner  NumberInputPorts=1
  IN_Message : PathCombiner  NumberInputPorts=1
  IN_MixedCarton1 : PathCombiner  NumberInputPorts=1
  IN_MixedPallet : PathCombiner  NumberInputPorts=1
  IN_Pallet : PathCombiner  NumberInputPorts=1
  Move : FRN_Library/Move
  OUTFlow_Signal : Replicate  NumberOutputPorts=2
  OUTFlow_Sort : OutputSwitch  NumberOutputPorts=5  SwitchingCriterion=From attribute  AttributeName=UoH
  OUT_Carton : OutputSwitch  NumberOutputPorts=1
  OUT_Each : OutputSwitch  NumberOutputPorts=1
  OUT_Message : OutputSwitch  NumberOutputPorts=1  SwitchingCriterion=Equiprobable  AttributeName=FlowSource
  OUT_MixedCarton : OutputSwitch  NumberOutputPorts=1
  OUT_MixedPallet : OutputSwitch  NumberOutputPorts=1
  OUT_Pallet : OutputSwitch  NumberOutputPorts=1
  IN_Carton_1 : PMIOPort  Port=1  Side=Left
  OUT_Carton_1 : PMIOPort  Port=2  Side=Right
  connections:
  INFlow_Signal/RConn2 -- Move/LConn1
  IN_MixedCarton1/RConn1 -- INFlow_Combine/LConn4
  IN_MixedPallet/RConn1 -- INFlow_Combine/LConn2
  OUTFlow_Sort/RConn4 -- OUT_MixedCarton/LConn1
  OUT_MixedPallet/LConn1 -- OUTFlow_Sort/RConn2
  Move/RConn2 -- OUT_Message/LConn1
  IN_Message/RConn1 -- Move/LConn2
  OUTFlow_Sort/RConn5 -- OUT_Each/LConn1
  OUTFlow_Sort/RConn3 -- OUT_Carton/LConn1
  OUT_Pallet/LConn1 -- OUTFlow_Sort/RConn1
  OUTFlow_Signal/RConn2 -- OUTFlow_Sort/LConn1
  IN_Each/RConn1 -- INFlow_Combine/LConn5
  IN_Carton/RConn1 -- INFlow_Combine/LConn3
  IN_Pallet/RConn1 -- INFlow_Combine/LConn1
  INFlow_Combine/RConn1 -- INFlow_Signal/LConn1
  OUTFlow_Signal/RConn1 -- Calculate_OUTFlow/RConn1
  Move/RConn1 -- OUTFlow_Signal/LConn1
  Calculate_OUTFlow/LConn2 -- FlowRecord/LConn2
  FlowRecord/LConn1 -- Calculate_OUTFlow/LConn1
  Calculate_INFlow/RConn2 -- FlowRecord/RConn2
  FlowRecord/RConn1 -- Calculate_INFlow/RConn1
  Calculate_INFlow/LConn1 -- INFlow_Signal/RConn1
  IN_Carton/LConn1 -- IN_Carton_1/RConn1
  OUT_Carton/RConn1 -- OUT_Carton_1/RConn1

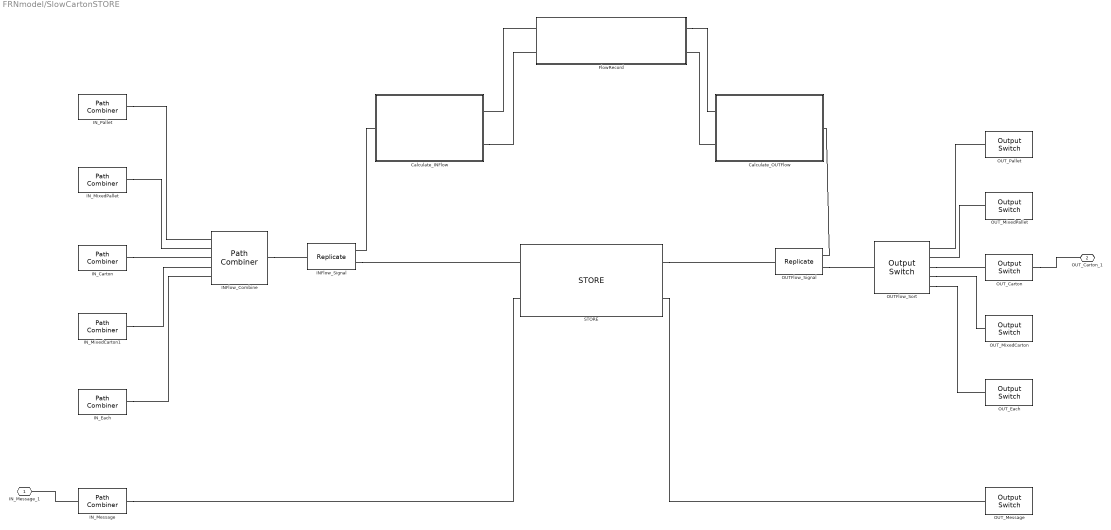
== system FRNmodel/SlowCartonSTORE ==
  Calculate_INFlow : Subsystem
  Calculate_OUTFlow : Subsystem
  FlowRecord : Subsystem
  INFlow_Combine : PathCombiner  NumberInputPorts=5
  INFlow_Signal : Replicate  NumberOutputPorts=2
  IN_Carton : PathCombiner  NumberInputPorts=1
  IN_Each : PathCombiner  NumberInputPorts=1
  IN_Message : PathCombiner  NumberInputPorts=1
  IN_MixedCarton1 : PathCombiner  NumberInputPorts=1
  IN_MixedPallet : PathCombiner  NumberInputPorts=1
  IN_Pallet : PathCombiner  NumberInputPorts=1
  OUTFlow_Signal : Replicate  NumberOutputPorts=2
  OUTFlow_Sort : OutputSwitch  NumberOutputPorts=5  SwitchingCriterion=From attribute  AttributeName=UoH
  OUT_Carton : OutputSwitch  NumberOutputPorts=1
  OUT_Each : OutputSwitch  NumberOutputPorts=1
  OUT_Message : OutputSwitch  NumberOutputPorts=1  SwitchingCriterion=Equiprobable  AttributeName=FlowSource
  OUT_MixedCarton : OutputSwitch  NumberOutputPorts=1
  OUT_MixedPallet : OutputSwitch  NumberOutputPorts=1
  OUT_Pallet : OutputSwitch  NumberOutputPorts=1
  STORE : FRN_Library/STORE
  IN_Message_1 : PMIOPort  Port=1  Side=Left
  OUT_Carton_1 : PMIOPort  Port=2  Side=Right
  connections:
  INFlow_Signal/RConn2 -- STORE/LConn1
  IN_MixedCarton1/RConn1 -- INFlow_Combine/LConn4
  IN_MixedPallet/RConn1 -- INFlow_Combine/LConn2
  OUTFlow_Sort/RConn4 -- OUT_MixedCarton/LConn1
  OUT_MixedPallet/LConn1 -- OUTFlow_Sort/RConn2
  STORE/RConn2 -- OUT_Message/LConn1
  IN_Message/RConn1 -- STORE/LConn2
  OUTFlow_Sort/RConn5 -- OUT_Each/LConn1
  OUTFlow_Sort/RConn3 -- OUT_Carton/LConn1
  OUT_Pallet/LConn1 -- OUTFlow_Sort/RConn1
  OUTFlow_Signal/RConn2 -- OUTFlow_Sort/LConn1
  IN_Each/RConn1 -- INFlow_Combine/LConn5
  IN_Carton/RConn1 -- INFlow_Combine/LConn3
  IN_Pallet/RConn1 -- INFlow_Combine/LConn1
  INFlow_Combine/RConn1 -- INFlow_Signal/LConn1
  OUTFlow_Signal/RConn1 -- Calculate_OUTFlow/RConn1
  STORE/RConn1 -- OUTFlow_Signal/LConn1
  Calculate_OUTFlow/LConn2 -- FlowRecord/LConn2
  FlowRecord/LConn1 -- Calculate_OUTFlow/LConn1
  Calculate_INFlow/RConn2 -- FlowRecord/RConn2
  FlowRecord/RConn1 -- Calculate_INFlow/RConn1
  Calculate_INFlow/LConn1 -- INFlow_Signal/RConn1
  IN_Message/LConn1 -- IN_Message_1/RConn1
  OUT_Carton/RConn1 -- OUT_Carton_1/RConn1

== system FRNmodel/FastCarton2MPassembly/Calculate_INFlow ==
  Calculate_INFlow : MATLAB Function  TreatAsAtomicUnit=on
  Entity Combiner : EntityCombiner  NumberInputPorts=2
  Entity Sink : EntitySink
  Entity Splitter : EntitySplitter  NumberOutputPorts=2
  FIFO Queue : FIFOQueue  Capacity=inf
  Get Attribute : GetAttribute  AttributeName=UoH|Quantity|INFlow  AttributeMissing=Error|Error|Error  AttributeDefaultValue=1|1|1  AttributeTreatAsVector=1|1|1  AttributeSendTiming=After entity departure|After entity departure|After entity departure  EvaluatedDefaultAttributeValue={[];[];[]}
      settings: OutputPortMap=o1,o2,o3
  Set Attribute : SetAttribute  AttributeName=INFlow  AttributeFrom=Signal port  EvaluatedAttributeValue={[]}
  Single Server : SingleServer  ServiceTime=0
  FlowRecord_IN : PMIOPort  Port=1  Side=Right
  FlowRecord_OUT : PMIOPort  Port=2  Side=Right
  INFlow_Signal : PMIOPort  Port=3  Side=Left
  wires:
  Get Attribute/3 -> Calculate_INFlow/3(INFlow)
  Get Attribute/2 -> Calculate_INFlow/2(Quantity)
  Calculate_INFlow/1(INFlow_return) -> Set Attribute/1
  Get Attribute/1 -> Calculate_INFlow/1(UoH)
  connections:
  FIFO Queue/RConn1 -- Entity Combiner/LConn2
  INFlow_Signal/RConn1 -- FIFO Queue/LConn1
  Entity Splitter/RConn2 -- Entity Sink/LConn1
  FlowRecord_IN/RConn1 -- Entity Combiner/LConn1
  FlowRecord_OUT/RConn1 -- Entity Splitter/RConn1
  Single Server/RConn1 -- Set Attribute/LConn1
  Get Attribute/RConn1 -- Single Server/LConn1
  Set Attribute/RConn1 -- Entity Splitter/LConn1
  Entity Combiner/RConn1 -- Get Attribute/LConn1

== system FRNmodel/FastCarton2MPassembly/Calculate_OUTFlow ==
  Calculate_OUTFlow : MATLAB Function  TreatAsAtomicUnit=on
  Entity Combiner : EntityCombiner  NumberInputPorts=2
  Entity Sink : EntitySink
  Entity Splitter : EntitySplitter  NumberOutputPorts=2
  FIFO Queue : FIFOQueue  Capacity=inf
  Get Attribute : GetAttribute  AttributeName=UoH|Quantity|OUTFlow  AttributeMissing=Error|Error|Error  AttributeDefaultValue=1|1|1  AttributeTreatAsVector=1|1|1  AttributeSendTiming=After entity departure|After entity departure|After entity departure  EvaluatedDefaultAttributeValue={[];[];[]}
      settings: OutputPortMap=o1,o2,o3
  Set Attribute : SetAttribute  AttributeName=OUTFlow  AttributeFrom=Signal port  EvaluatedAttributeValue={[]}
  Single Server : SingleServer  ServiceTime=0
  FlowRecord_IN : PMIOPort  Port=1  Side=Left
  FlowRecord_OUT : PMIOPort  Port=2  Side=Left
  OUTFlow_Signal : PMIOPort  Port=3  Side=Right
  wires:
  Get Attribute/3 -> Calculate_OUTFlow/3(OUTFlow)
  Get Attribute/2 -> Calculate_OUTFlow/2(Quantity)
  Calculate_OUTFlow/1(OUTFlow_return) -> Set Attribute/1
  Get Attribute/1 -> Calculate_OUTFlow/1(UoH)
  connections:
  Entity Splitter/RConn2 -- Entity Sink/LConn1
  FIFO Queue/RConn1 -- Entity Combiner/LConn2
  OUTFlow_Signal/RConn1 -- FIFO Queue/LConn1
  FlowRecord_IN/RConn1 -- Entity Combiner/LConn1
  FlowRecord_OUT/RConn1 -- Entity Splitter/RConn1
  Single Server/RConn1 -- Set Attribute/LConn1
  Get Attribute/RConn1 -- Single Server/LConn1
  Set Attribute/RConn1 -- Entity Splitter/LConn1
  Entity Combiner/RConn1 -- Get Attribute/LConn1

== system FRNmodel/FastCarton2MPassembly/FlowRecord ==
  FIFO Queue : FIFOQueue
  FlowRecord : TimeBasedFunctionCallGenerator  EventGenerationMode=Only at simulation start
  Get Attribute : GetAttribute  AttributeName=OUTFlow|INFlow  AttributeMissing=Error|Error  AttributeDefaultValue=1|1  AttributeTreatAsVector=1|1  AttributeSendTiming=After entity departure|After entity departure  EvaluatedDefaultAttributeValue={[];[]}
      settings: OutputPortMap=o1,o2
  INFlow_Metric : simeventslib/SimEvents Sinks/Discrete Event Signal to Workspace  VariableName=INFlow_Metric_FastCarton2MPassembly  SaveFormat=Structure With Time  isMonitorOnly=off  isRecordIC=off
  Initialize_FlowRecord : SetAttribute  AttributeName=INFlow|OUTFlow  AttributeFrom=Dialog|Dialog  AttributeValue=[0 0 0 0 0]|[0 0 0 0 0]  AttributeTreatAsVector=1|1  EvaluatedAttributeValue={[0 0 0 0 0];[0 0 0 0 0]}
  New_FlowRecord : EventBasedEntityGenerator  GenerateEntitiesUpon=Function call from port fcn
  OUTFlow_Metric : simeventslib/SimEvents Sinks/Discrete Event Signal to Workspace  VariableName=OUTFlow_Metric_FastCarton2MPassembly  SaveFormat=Structure With Time  isMonitorOnly=off  isRecordIC=off
  Output Switch : OutputSwitch  NumberOutputPorts=2
  Path Combiner1 : PathCombiner
  TO_INFlow : PMIOPort  Port=1  Side=Right
  TO_OUTFlow : PMIOPort  Port=2  Side=Left
  FROM_INFlow : PMIOPort  Port=3  Side=Right
  FROM_OUTFlow : PMIOPort  Port=4  Side=Left
  wires:
  Get Attribute/2 -> INFlow_Metric/1
  Get Attribute/1 -> OUTFlow_Metric/1
  FlowRecord/1 -> New_FlowRecord/1
  connections:
  Get Attribute/RConn1 -- FIFO Queue/LConn1
  Path Combiner1/RConn1 -- Get Attribute/LConn1
  FROM_OUTFlow/RConn1 -- Path Combiner1/LConn3
  FROM_INFlow/RConn1 -- Path Combiner1/LConn2
  TO_OUTFlow/RConn1 -- Output Switch/RConn2
  TO_INFlow/RConn1 -- Output Switch/RConn1
  Initialize_FlowRecord/RConn1 -- Path Combiner1/LConn1
  New_FlowRecord/RConn1 -- Initialize_FlowRecord/LConn1
  Output Switch/LConn1 -- FIFO Queue/RConn1

== system FRNmodel/FastCartonSTORE/Calculate_INFlow ==
  Calculate_INFlow : MATLAB Function  TreatAsAtomicUnit=on
  Entity Combiner : EntityCombiner  NumberInputPorts=2
  Entity Sink : EntitySink
  Entity Splitter : EntitySplitter  NumberOutputPorts=2
  FIFO Queue : FIFOQueue  Capacity=inf
  Get Attribute : GetAttribute  AttributeName=UoH|Quantity|INFlow  AttributeMissing=Error|Error|Error  AttributeDefaultValue=1|1|1  AttributeTreatAsVector=1|1|1  AttributeSendTiming=After entity departure|After entity departure|After entity departure  EvaluatedDefaultAttributeValue={[];[];[]}
      settings: OutputPortMap=o1,o2,o3
  Set Attribute : SetAttribute  AttributeName=INFlow  AttributeFrom=Signal port  EvaluatedAttributeValue={[]}
  Single Server : SingleServer  ServiceTime=0
  FlowRecord_IN : PMIOPort  Port=1  Side=Right
  FlowRecord_OUT : PMIOPort  Port=2  Side=Right
  INFlow_Signal : PMIOPort  Port=3  Side=Left
  wires:
  Get Attribute/3 -> Calculate_INFlow/3(INFlow)
  Get Attribute/2 -> Calculate_INFlow/2(Quantity)
  Calculate_INFlow/1(INFlow_return) -> Set Attribute/1
  Get Attribute/1 -> Calculate_INFlow/1(UoH)
  connections:
  FIFO Queue/RConn1 -- Entity Combiner/LConn2
  INFlow_Signal/RConn1 -- FIFO Queue/LConn1
  Entity Splitter/RConn2 -- Entity Sink/LConn1
  FlowRecord_IN/RConn1 -- Entity Combiner/LConn1
  FlowRecord_OUT/RConn1 -- Entity Splitter/RConn1
  Single Server/RConn1 -- Set Attribute/LConn1
  Get Attribute/RConn1 -- Single Server/LConn1
  Set Attribute/RConn1 -- Entity Splitter/LConn1
  Entity Combiner/RConn1 -- Get Attribute/LConn1

== system FRNmodel/FastCartonSTORE/Calculate_OUTFlow ==
  Calculate_OUTFlow : MATLAB Function  TreatAsAtomicUnit=on
  Entity Combiner : EntityCombiner  NumberInputPorts=2
  Entity Sink : EntitySink
  Entity Splitter : EntitySplitter  NumberOutputPorts=2
  FIFO Queue : FIFOQueue  Capacity=inf
  Get Attribute : GetAttribute  AttributeName=UoH|Quantity|OUTFlow  AttributeMissing=Error|Error|Error  AttributeDefaultValue=1|1|1  AttributeTreatAsVector=1|1|1  AttributeSendTiming=After entity departure|After entity departure|After entity departure  EvaluatedDefaultAttributeValue={[];[];[]}
      settings: OutputPortMap=o1,o2,o3
  Set Attribute : SetAttribute  AttributeName=OUTFlow  AttributeFrom=Signal port  EvaluatedAttributeValue={[]}
  Single Server : SingleServer  ServiceTime=0
  FlowRecord_IN : PMIOPort  Port=1  Side=Left
  FlowRecord_OUT : PMIOPort  Port=2  Side=Left
  OUTFlow_Signal : PMIOPort  Port=3  Side=Right
  wires:
  Get Attribute/3 -> Calculate_OUTFlow/3(OUTFlow)
  Get Attribute/2 -> Calculate_OUTFlow/2(Quantity)
  Calculate_OUTFlow/1(OUTFlow_return) -> Set Attribute/1
  Get Attribute/1 -> Calculate_OUTFlow/1(UoH)
  connections:
  Entity Splitter/RConn2 -- Entity Sink/LConn1
  FIFO Queue/RConn1 -- Entity Combiner/LConn2
  OUTFlow_Signal/RConn1 -- FIFO Queue/LConn1
  FlowRecord_IN/RConn1 -- Entity Combiner/LConn1
  FlowRecord_OUT/RConn1 -- Entity Splitter/RConn1
  Single Server/RConn1 -- Set Attribute/LConn1
  Get Attribute/RConn1 -- Single Server/LConn1
  Set Attribute/RConn1 -- Entity Splitter/LConn1
  Entity Combiner/RConn1 -- Get Attribute/LConn1

== system FRNmodel/FastCartonSTORE/FlowRecord ==
  FIFO Queue : FIFOQueue
  FlowRecord : TimeBasedFunctionCallGenerator  EventGenerationMode=Only at simulation start
  Get Attribute : GetAttribute  AttributeName=OUTFlow|INFlow  AttributeMissing=Error|Error  AttributeDefaultValue=1|1  AttributeTreatAsVector=1|1  AttributeSendTiming=After entity departure|After entity departure  EvaluatedDefaultAttributeValue={[];[]}
      settings: OutputPortMap=o1,o2
  INFlow_Metric : simeventslib/SimEvents Sinks/Discrete Event Signal to Workspace  VariableName=INFlow_Metric_FastCartonSTORE  SaveFormat=Structure With Time  isMonitorOnly=off  isRecordIC=off
  Initialize_FlowRecord : SetAttribute  AttributeName=INFlow|OUTFlow  AttributeFrom=Dialog|Dialog  AttributeValue=[0 0 0 0 0]|[0 0 0 0 0]  AttributeTreatAsVector=1|1  EvaluatedAttributeValue={[0 0 0 0 0];[0 0 0 0 0]}
  New_FlowRecord : EventBasedEntityGenerator  GenerateEntitiesUpon=Function call from port fcn
  OUTFlow_Metric : simeventslib/SimEvents Sinks/Discrete Event Signal to Workspace  VariableName=OUTFlow_Metric_FastCartonSTORE  SaveFormat=Structure With Time  isMonitorOnly=off  isRecordIC=off
  Output Switch : OutputSwitch  NumberOutputPorts=2
  Path Combiner1 : PathCombiner
  TO_INFlow : PMIOPort  Port=1  Side=Right
  TO_OUTFlow : PMIOPort  Port=2  Side=Left
  FROM_INFlow : PMIOPort  Port=3  Side=Right
  FROM_OUTFlow : PMIOPort  Port=4  Side=Left
  wires:
  Get Attribute/2 -> INFlow_Metric/1
  Get Attribute/1 -> OUTFlow_Metric/1
  FlowRecord/1 -> New_FlowRecord/1
  connections:
  Get Attribute/RConn1 -- FIFO Queue/LConn1
  Path Combiner1/RConn1 -- Get Attribute/LConn1
  FROM_OUTFlow/RConn1 -- Path Combiner1/LConn3
  FROM_INFlow/RConn1 -- Path Combiner1/LConn2
  TO_OUTFlow/RConn1 -- Output Switch/RConn2
  TO_INFlow/RConn1 -- Output Switch/RConn1
  Initialize_FlowRecord/RConn1 -- Path Combiner1/LConn1
  New_FlowRecord/RConn1 -- Initialize_FlowRecord/LConn1
  Output Switch/LConn1 -- FIFO Queue/RConn1

== system FRNmodel/HeavyCarton2MPassembly/Calculate_INFlow ==
  Calculate_INFlow : MATLAB Function  TreatAsAtomicUnit=on
  Entity Combiner : EntityCombiner  NumberInputPorts=2
  Entity Sink : EntitySink
  Entity Splitter : EntitySplitter  NumberOutputPorts=2
  FIFO Queue : FIFOQueue  Capacity=inf
  Get Attribute : GetAttribute  AttributeName=UoH|Quantity|INFlow  AttributeMissing=Error|Error|Error  AttributeDefaultValue=1|1|1  AttributeTreatAsVector=1|1|1  AttributeSendTiming=After entity departure|After entity departure|After entity departure  EvaluatedDefaultAttributeValue={[];[];[]}
      settings: OutputPortMap=o1,o2,o3
  Set Attribute : SetAttribute  AttributeName=INFlow  AttributeFrom=Signal port  EvaluatedAttributeValue={[]}
  Single Server : SingleServer  ServiceTime=0
  FlowRecord_IN : PMIOPort  Port=1  Side=Right
  FlowRecord_OUT : PMIOPort  Port=2  Side=Right
  INFlow_Signal : PMIOPort  Port=3  Side=Left
  wires:
  Get Attribute/3 -> Calculate_INFlow/3(INFlow)
  Get Attribute/2 -> Calculate_INFlow/2(Quantity)
  Calculate_INFlow/1(INFlow_return) -> Set Attribute/1
  Get Attribute/1 -> Calculate_INFlow/1(UoH)
  connections:
  FIFO Queue/RConn1 -- Entity Combiner/LConn2
  INFlow_Signal/RConn1 -- FIFO Queue/LConn1
  Entity Splitter/RConn2 -- Entity Sink/LConn1
  FlowRecord_IN/RConn1 -- Entity Combiner/LConn1
  FlowRecord_OUT/RConn1 -- Entity Splitter/RConn1
  Single Server/RConn1 -- Set Attribute/LConn1
  Get Attribute/RConn1 -- Single Server/LConn1
  Set Attribute/RConn1 -- Entity Splitter/LConn1
  Entity Combiner/RConn1 -- Get Attribute/LConn1

== system FRNmodel/HeavyCarton2MPassembly/Calculate_OUTFlow ==
  Calculate_OUTFlow : MATLAB Function  TreatAsAtomicUnit=on
  Entity Combiner : EntityCombiner  NumberInputPorts=2
  Entity Sink : EntitySink
  Entity Splitter : EntitySplitter  NumberOutputPorts=2
  FIFO Queue : FIFOQueue  Capacity=inf
  Get Attribute : GetAttribute  AttributeName=UoH|Quantity|OUTFlow  AttributeMissing=Error|Error|Error  AttributeDefaultValue=1|1|1  AttributeTreatAsVector=1|1|1  AttributeSendTiming=After entity departure|After entity departure|After entity departure  EvaluatedDefaultAttributeValue={[];[];[]}
      settings: OutputPortMap=o1,o2,o3
  Set Attribute : SetAttribute  AttributeName=OUTFlow  AttributeFrom=Signal port  EvaluatedAttributeValue={[]}
  Single Server : SingleServer  ServiceTime=0
  FlowRecord_IN : PMIOPort  Port=1  Side=Left
  FlowRecord_OUT : PMIOPort  Port=2  Side=Left
  OUTFlow_Signal : PMIOPort  Port=3  Side=Right
  wires:
  Get Attribute/3 -> Calculate_OUTFlow/3(OUTFlow)
  Get Attribute/2 -> Calculate_OUTFlow/2(Quantity)
  Calculate_OUTFlow/1(OUTFlow_return) -> Set Attribute/1
  Get Attribute/1 -> Calculate_OUTFlow/1(UoH)
  connections:
  Entity Splitter/RConn2 -- Entity Sink/LConn1
  FIFO Queue/RConn1 -- Entity Combiner/LConn2
  OUTFlow_Signal/RConn1 -- FIFO Queue/LConn1
  FlowRecord_IN/RConn1 -- Entity Combiner/LConn1
  FlowRecord_OUT/RConn1 -- Entity Splitter/RConn1
  Single Server/RConn1 -- Set Attribute/LConn1
  Get Attribute/RConn1 -- Single Server/LConn1
  Set Attribute/RConn1 -- Entity Splitter/LConn1
  Entity Combiner/RConn1 -- Get Attribute/LConn1

== system FRNmodel/HeavyCarton2MPassembly/FlowRecord ==
  FIFO Queue : FIFOQueue
  FlowRecord : TimeBasedFunctionCallGenerator  EventGenerationMode=Only at simulation start
  Get Attribute : GetAttribute  AttributeName=OUTFlow|INFlow  AttributeMissing=Error|Error  AttributeDefaultValue=1|1  AttributeTreatAsVector=1|1  AttributeSendTiming=After entity departure|After entity departure  EvaluatedDefaultAttributeValue={[];[]}
      settings: OutputPortMap=o1,o2
  INFlow_Metric : simeventslib/SimEvents Sinks/Discrete Event Signal to Workspace  VariableName=INFlow_Metric_HeavyCarton2MPassembly  SaveFormat=Structure With Time  isMonitorOnly=off  isRecordIC=off
  Initialize_FlowRecord : SetAttribute  AttributeName=INFlow|OUTFlow  AttributeFrom=Dialog|Dialog  AttributeValue=[0 0 0 0 0]|[0 0 0 0 0]  AttributeTreatAsVector=1|1  EvaluatedAttributeValue={[0 0 0 0 0];[0 0 0 0 0]}
  New_FlowRecord : EventBasedEntityGenerator  GenerateEntitiesUpon=Function call from port fcn
  OUTFlow_Metric : simeventslib/SimEvents Sinks/Discrete Event Signal to Workspace  VariableName=OUTFlow_Metric_HeavyCarton2MPassembly  SaveFormat=Structure With Time  isMonitorOnly=off  isRecordIC=off
  Output Switch : OutputSwitch  NumberOutputPorts=2
  Path Combiner1 : PathCombiner
  TO_INFlow : PMIOPort  Port=1  Side=Right
  TO_OUTFlow : PMIOPort  Port=2  Side=Left
  FROM_INFlow : PMIOPort  Port=3  Side=Right
  FROM_OUTFlow : PMIOPort  Port=4  Side=Left
  wires:
  Get Attribute/2 -> INFlow_Metric/1
  Get Attribute/1 -> OUTFlow_Metric/1
  FlowRecord/1 -> New_FlowRecord/1
  connections:
  Get Attribute/RConn1 -- FIFO Queue/LConn1
  Path Combiner1/RConn1 -- Get Attribute/LConn1
  FROM_OUTFlow/RConn1 -- Path Combiner1/LConn3
  FROM_INFlow/RConn1 -- Path Combiner1/LConn2
  TO_OUTFlow/RConn1 -- Output Switch/RConn2
  TO_INFlow/RConn1 -- Output Switch/RConn1
  Initialize_FlowRecord/RConn1 -- Path Combiner1/LConn1
  New_FlowRecord/RConn1 -- Initialize_FlowRecord/LConn1
  Output Switch/LConn1 -- FIFO Queue/RConn1

== system FRNmodel/HeavyCartonSTORE/Calculate_INFlow ==
  Calculate_INFlow : MATLAB Function  TreatAsAtomicUnit=on
  Entity Combiner : EntityCombiner  NumberInputPorts=2
  Entity Sink : EntitySink
  Entity Splitter : EntitySplitter  NumberOutputPorts=2
  FIFO Queue : FIFOQueue  Capacity=inf
  Get Attribute : GetAttribute  AttributeName=UoH|Quantity|INFlow  AttributeMissing=Error|Error|Error  AttributeDefaultValue=1|1|1  AttributeTreatAsVector=1|1|1  AttributeSendTiming=After entity departure|After entity departure|After entity departure  EvaluatedDefaultAttributeValue={[];[];[]}
      settings: OutputPortMap=o1,o2,o3
  Set Attribute : SetAttribute  AttributeName=INFlow  AttributeFrom=Signal port  EvaluatedAttributeValue={[]}
  Single Server : SingleServer  ServiceTime=0
  FlowRecord_IN : PMIOPort  Port=1  Side=Right
  FlowRecord_OUT : PMIOPort  Port=2  Side=Right
  INFlow_Signal : PMIOPort  Port=3  Side=Left
  wires:
  Get Attribute/3 -> Calculate_INFlow/3(INFlow)
  Get Attribute/2 -> Calculate_INFlow/2(Quantity)
  Calculate_INFlow/1(INFlow_return) -> Set Attribute/1
  Get Attribute/1 -> Calculate_INFlow/1(UoH)
  connections:
  FIFO Queue/RConn1 -- Entity Combiner/LConn2
  INFlow_Signal/RConn1 -- FIFO Queue/LConn1
  Entity Splitter/RConn2 -- Entity Sink/LConn1
  FlowRecord_IN/RConn1 -- Entity Combiner/LConn1
  FlowRecord_OUT/RConn1 -- Entity Splitter/RConn1
  Single Server/RConn1 -- Set Attribute/LConn1
  Get Attribute/RConn1 -- Single Server/LConn1
  Set Attribute/RConn1 -- Entity Splitter/LConn1
  Entity Combiner/RConn1 -- Get Attribute/LConn1

== system FRNmodel/HeavyCartonSTORE/Calculate_OUTFlow ==
  Calculate_OUTFlow : MATLAB Function  TreatAsAtomicUnit=on
  Entity Combiner : EntityCombiner  NumberInputPorts=2
  Entity Sink : EntitySink
  Entity Splitter : EntitySplitter  NumberOutputPorts=2
  FIFO Queue : FIFOQueue  Capacity=inf
  Get Attribute : GetAttribute  AttributeName=UoH|Quantity|OUTFlow  AttributeMissing=Error|Error|Error  AttributeDefaultValue=1|1|1  AttributeTreatAsVector=1|1|1  AttributeSendTiming=After entity departure|After entity departure|After entity departure  EvaluatedDefaultAttributeValue={[];[];[]}
      settings: OutputPortMap=o1,o2,o3
  Set Attribute : SetAttribute  AttributeName=OUTFlow  AttributeFrom=Signal port  EvaluatedAttributeValue={[]}
  Single Server : SingleServer  ServiceTime=0
  FlowRecord_IN : PMIOPort  Port=1  Side=Left
  FlowRecord_OUT : PMIOPort  Port=2  Side=Left
  OUTFlow_Signal : PMIOPort  Port=3  Side=Right
  wires:
  Get Attribute/3 -> Calculate_OUTFlow/3(OUTFlow)
  Get Attribute/2 -> Calculate_OUTFlow/2(Quantity)
  Calculate_OUTFlow/1(OUTFlow_return) -> Set Attribute/1
  Get Attribute/1 -> Calculate_OUTFlow/1(UoH)
  connections:
  Entity Splitter/RConn2 -- Entity Sink/LConn1
  FIFO Queue/RConn1 -- Entity Combiner/LConn2
  OUTFlow_Signal/RConn1 -- FIFO Queue/LConn1
  FlowRecord_IN/RConn1 -- Entity Combiner/LConn1
  FlowRecord_OUT/RConn1 -- Entity Splitter/RConn1
  Single Server/RConn1 -- Set Attribute/LConn1
  Get Attribute/RConn1 -- Single Server/LConn1
  Set Attribute/RConn1 -- Entity Splitter/LConn1
  Entity Combiner/RConn1 -- Get Attribute/LConn1

== system FRNmodel/HeavyCartonSTORE/FlowRecord ==
  FIFO Queue : FIFOQueue
  FlowRecord : TimeBasedFunctionCallGenerator  EventGenerationMode=Only at simulation start
  Get Attribute : GetAttribute  AttributeName=OUTFlow|INFlow  AttributeMissing=Error|Error  AttributeDefaultValue=1|1  AttributeTreatAsVector=1|1  AttributeSendTiming=After entity departure|After entity departure  EvaluatedDefaultAttributeValue={[];[]}
      settings: OutputPortMap=o1,o2
  INFlow_Metric : simeventslib/SimEvents Sinks/Discrete Event Signal to Workspace  VariableName=INFlow_Metric_HeavyCartonSTORE  SaveFormat=Structure With Time  isMonitorOnly=off  isRecordIC=off
  Initialize_FlowRecord : SetAttribute  AttributeName=INFlow|OUTFlow  AttributeFrom=Dialog|Dialog  AttributeValue=[0 0 0 0 0]|[0 0 0 0 0]  AttributeTreatAsVector=1|1  EvaluatedAttributeValue={[0 0 0 0 0];[0 0 0 0 0]}
  New_FlowRecord : EventBasedEntityGenerator  GenerateEntitiesUpon=Function call from port fcn
  OUTFlow_Metric : simeventslib/SimEvents Sinks/Discrete Event Signal to Workspace  VariableName=OUTFlow_Metric_HeavyCartonSTORE  SaveFormat=Structure With Time  isMonitorOnly=off  isRecordIC=off
  Output Switch : OutputSwitch  NumberOutputPorts=2
  Path Combiner1 : PathCombiner
  TO_INFlow : PMIOPort  Port=1  Side=Right
  TO_OUTFlow : PMIOPort  Port=2  Side=Left
  FROM_INFlow : PMIOPort  Port=3  Side=Right
  FROM_OUTFlow : PMIOPort  Port=4  Side=Left
  wires:
  Get Attribute/2 -> INFlow_Metric/1
  Get Attribute/1 -> OUTFlow_Metric/1
  FlowRecord/1 -> New_FlowRecord/1
  connections:
  Get Attribute/RConn1 -- FIFO Queue/LConn1
  Path Combiner1/RConn1 -- Get Attribute/LConn1
  FROM_OUTFlow/RConn1 -- Path Combiner1/LConn3
  FROM_INFlow/RConn1 -- Path Combiner1/LConn2
  TO_OUTFlow/RConn1 -- Output Switch/RConn2
  TO_INFlow/RConn1 -- Output Switch/RConn1
  Initialize_FlowRecord/RConn1 -- Path Combiner1/LConn1
  New_FlowRecord/RConn1 -- Initialize_FlowRecord/LConn1
  Output Switch/LConn1 -- FIFO Queue/RConn1

== system FRNmodel/LTL/Calculate_INFlow ==
  Calculate_INFlow : MATLAB Function  TreatAsAtomicUnit=on
  Entity Combiner : EntityCombiner  NumberInputPorts=2
  Entity Sink : EntitySink
  Entity Splitter : EntitySplitter  NumberOutputPorts=2
  FIFO Queue : FIFOQueue  Capacity=inf
  Get Attribute : GetAttribute  AttributeName=UoH|Quantity|INFlow  AttributeMissing=Error|Error|Error  AttributeDefaultValue=1|1|1  AttributeTreatAsVector=1|1|1  AttributeSendTiming=After entity departure|After entity departure|After entity departure  EvaluatedDefaultAttributeValue={[];[];[]}
      settings: OutputPortMap=o1,o2,o3
  Set Attribute : SetAttribute  AttributeName=INFlow  AttributeFrom=Signal port  EvaluatedAttributeValue={[]}
  Single Server : SingleServer  ServiceTime=0
  FlowRecord_IN : PMIOPort  Port=1  Side=Right
  FlowRecord_OUT : PMIOPort  Port=2  Side=Right
  INFlow_Signal : PMIOPort  Port=3  Side=Left
  wires:
  Get Attribute/3 -> Calculate_INFlow/3(INFlow)
  Get Attribute/2 -> Calculate_INFlow/2(Quantity)
  Calculate_INFlow/1(INFlow_return) -> Set Attribute/1
  Get Attribute/1 -> Calculate_INFlow/1(UoH)
  connections:
  FIFO Queue/RConn1 -- Entity Combiner/LConn2
  INFlow_Signal/RConn1 -- FIFO Queue/LConn1
  Entity Splitter/RConn2 -- Entity Sink/LConn1
  FlowRecord_IN/RConn1 -- Entity Combiner/LConn1
  FlowRecord_OUT/RConn1 -- Entity Splitter/RConn1
  Single Server/RConn1 -- Set Attribute/LConn1
  Get Attribute/RConn1 -- Single Server/LConn1
  Set Attribute/RConn1 -- Entity Splitter/LConn1
  Entity Combiner/RConn1 -- Get Attribute/LConn1
